simulink model "LQR"  (R2025b)
settings: Solver=VariableStepAuto  StartTime=0.0  StopTime=10.0  RelTol=1e-3
values from neighbouring files (symbols this model uses):
  A = double(subs(A_sym, [x; u], [x_star; u_star]))    [EsercitazioneEsame.m]
  B = [0; 0]    [Controllo_Avanzato_1.m]    (also in EsercitazioneEsame.m = double(subs(B_sym, [x; u], [x_star; u_star])))
  C = eye(2)    [Controllo_Avanzato_1.m]    (also in EsercitazioneEsame.m = eye(n))
  D = 0    [Controllo_Avanzato_1.m]    (also in EsercitazioneEsame.m = zeros(n, size(B, 2)))
undefined symbols (not defined in the file or in its folder): h0, Kint1, Kint2
settings Model: Creator=inggi  LastModifiedBy=inggi

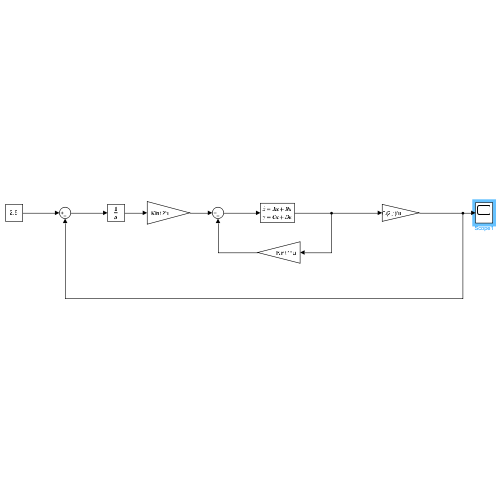
[thumbnail: Simulink's stored preview of the top-level diagram]
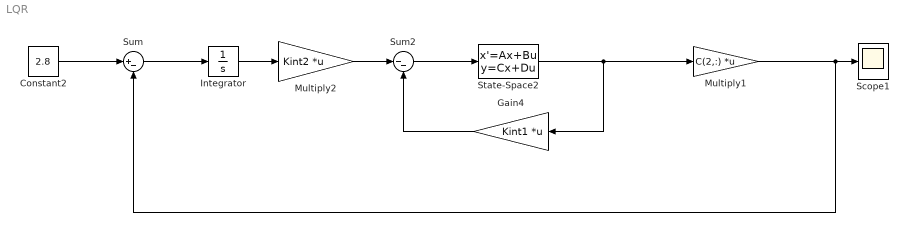
== system LQR ==
  Constant2 : Constant  Value=2.8
  Gain4 : Gain  Gain=Kint1  Multiplication=Matrix(K*u)
  Integrator : Integrator
  Multiply1 : Gain  Gain=C(2,:)  Multiplication=Matrix(K*u)
  Multiply2 : Gain  Gain=Kint2  Multiplication=Matrix(K*u)
  Scope1 : Scope
      settings: ActiveDisplayYMinimum=-0.14793270427814242  ActiveDisplayYMaximum=3.1275314942639492
  State-Space2 : StateSpace  A=A  B=B  C=C  D=D  InitialCondition=h0
  Sum : Sum  Inputs=|+-
  Sum2 : Sum  Inputs=|--
  wires:
  Multiply2/1 -> Sum2/1
  State-Space2/1 -> Multiply1/1, Gain4/1
  Multiply1/1 -> Sum/2, Scope1/1
  Sum2/1 -> State-Space2/1
  Integrator/1 -> Multiply2/1
  Sum/1 -> Integrator/1
  Gain4/1 -> Sum2/2
  Constant2/1 -> Sum/1
